simulink model "BicyclePeterCorke"  (R2021a)
settings: Solver=VariableStepAuto  StartTime=0.0  StopTime=10.0  RelTol=1e-3
values from neighbouring files (symbols this model uses):
  accelLim = 1    [BicyclePeterCorkeP2PSetup.m]    (also in BicyclePeterCorkeSetup.m)
  goalCoord = [5 5]    [BicyclePeterCorkeP2PSetup.m]    (also in BicyclePeterCorkeSetup.m)
  initCoord = [8 5 pi/2]    [BicyclePeterCorkeP2PSetup.m]    (also in BicyclePeterCorkeSetup.m)
  speedLim = 1    [BicyclePeterCorkeP2PSetup.m]    (also in BicyclePeterCorkeSetup.m)
  steerLim = 1    [BicyclePeterCorkeP2PSetup.m]    (also in BicyclePeterCorkeSetup.m)
  wheelBase = 1    [BicyclePeterCorkeP2PSetup.m]    (also in BicyclePeterCorkeSetup.m)
libraries: simulink x1
settings Model: Creator=guyot  LastModifiedBy=guyot

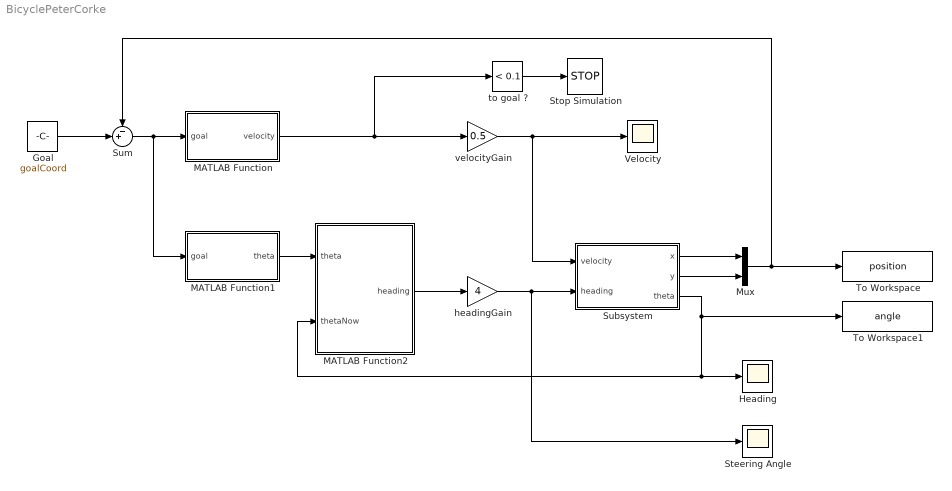
== system BicyclePeterCorke ==
  Goal : Constant  Value=goalCoord
  Heading : Scope
  MATLAB Function : MATLAB Function  TreatAsAtomicUnit=on
  MATLAB Function1 : MATLAB Function  TreatAsAtomicUnit=on
  MATLAB Function2 : MATLAB Function  TreatAsAtomicUnit=on
  Mux : Mux  Inputs=2
  Steering Angle : Scope
  Stop Simulation : Stop
  Subsystem : Subsystem
  Sum : Sum  Inputs=-+|
  To Workspace : ToWorkspace  VariableName=position  SaveFormat=Timeseries  SampleTime=-1
  To Workspace1 : ToWorkspace  VariableName=angle  SaveFormat=Timeseries  SampleTime=-1
  Velocity : Scope
  headingGain : Gain  Gain=4
  to goal ? : simulink/Logic and Bit Operations/Compare To Constant  relop=<  const=0.1  OutDataTypeStr=boolean
  velocityGain : Gain  Gain=0.5
  wires:
  Goal/1 -> Sum/2
  Sum/1 -> MATLAB Function1/1(goal), MATLAB Function/1(goal)
  MATLAB Function/1(velocity) -> to goal ?/1, velocityGain/1
  velocityGain/1 -> Subsystem/1(velocity), Velocity/1
  MATLAB Function1/1(theta) -> MATLAB Function2/1(theta)
  MATLAB Function2/1(heading) -> headingGain/1
  headingGain/1 -> Steering Angle/1, Subsystem/2(heading)
  Subsystem/1(x) -> Mux/1
  Subsystem/2(y) -> Mux/2
  Mux/1 -> To Workspace/1, Sum/1
  Subsystem/3(theta) -> To Workspace1/1, Heading/1, MATLAB Function2/2(thetaNow)
  to goal ?/1 -> Stop Simulation/1

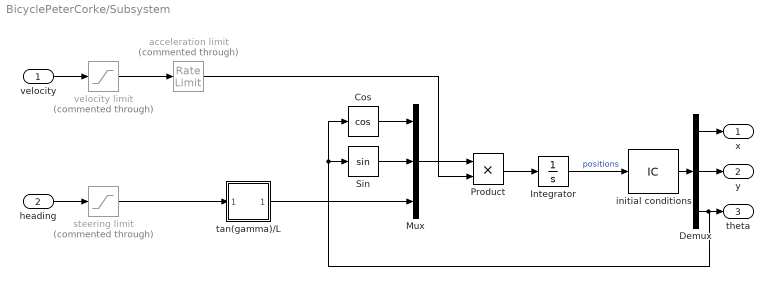
== system BicyclePeterCorke/Subsystem ==
  velocity : Inport
  heading : Inport  Port=2
  Cos : Trigonometry  Operator=cos
  Demux : Demux  Outputs=3
  Integrator : Integrator
  Mux : Mux  Inputs=3
  Product : Product
  Sin : Trigonometry
  acceleration limit : RateLimiter  Commented=through  RisingSlewLimit=accelLim  FallingSlewLimit=-accelLim  SampleTimeMode=inherited
  initial conditions : InitialCondition  Value=initCoord
  steering limit : Saturate  Commented=through  UpperLimit=steerLim  LowerLimit=-steerLim
  tan(gamma)/L : Subsystem
  velocity limit : Saturate  Commented=through  UpperLimit=speedLim  LowerLimit=-speedLim
  x : Outport
  y : Outport  Port=2
  theta : Outport  Port=3
  wires:
  velocity/1 -> velocity limit/1
  velocity limit/1 -> acceleration limit/1
  heading/1 -> steering limit/1
  steering limit/1 -> tan(gamma)/L/1(In1)
  tan(gamma)/L/1(Out1) -> Mux/3
  Mux/1 -> Product/1
  acceleration limit/1 -> Product/2
  Product/1 -> Integrator/1
  Integrator/1 -> initial conditions/1  "positions"
  Demux/3 -> Cos/1, Sin/1, theta/1
  Demux/1 -> x/1
  Demux/2 -> y/1
  Cos/1 -> Mux/1
  Sin/1 -> Mux/2
  initial conditions/1 -> Demux/1

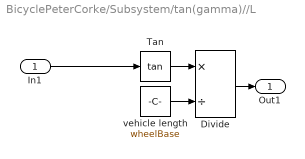
== system BicyclePeterCorke/Subsystem/tan(gamma)//L ==
  In1 : Inport
  Divide : Product  Inputs=*/
  Tan : Trigonometry  Operator=tan
  vehicle length : Constant  Value=wheelBase
  Out1 : Outport
  wires:
  Tan/1 -> Divide/1
  vehicle length/1 -> Divide/2
  In1/1 -> Tan/1
  Divide/1 -> Out1/1

== matlab function BicyclePeterCorke/MATLAB Function ==
  data: goal input; velocity output
function velocity = speedGoal(goal)

velocity = sqrt(goal(1)^2+goal(2)^2);

== matlab function BicyclePeterCorke/MATLAB Function2 ==
  data: theta input; heading output; thetaNow input
function heading = gammaGoal(theta, thetaNow)

heading = angdiff(theta, thetaNow);

== matlab function BicyclePeterCorke/MATLAB Function1 ==
  data: goal input; theta output
function theta = goalAngle(goal)

theta = atan2(goal(2),goal(1));
